simulink model "sampleModel1404"  (R2023a)
settings: Solver=VariableStepAuto  StartTime=0.0  StopTime=10.0  RelTol=1e-3
libraries: simulink x5, hdlsllib x1
settings Model: Creator=user1  LastModifiedBy=user1

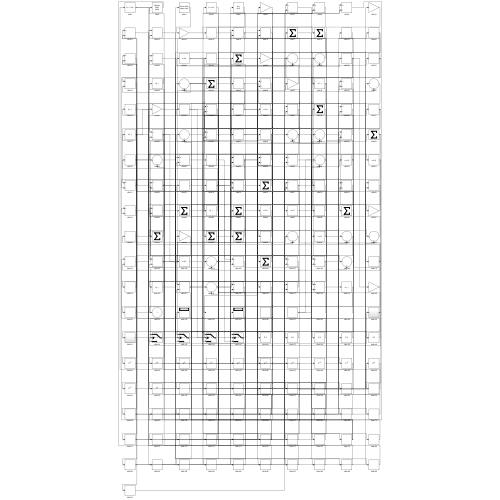
[thumbnail: Simulink's stored preview of the top-level diagram]
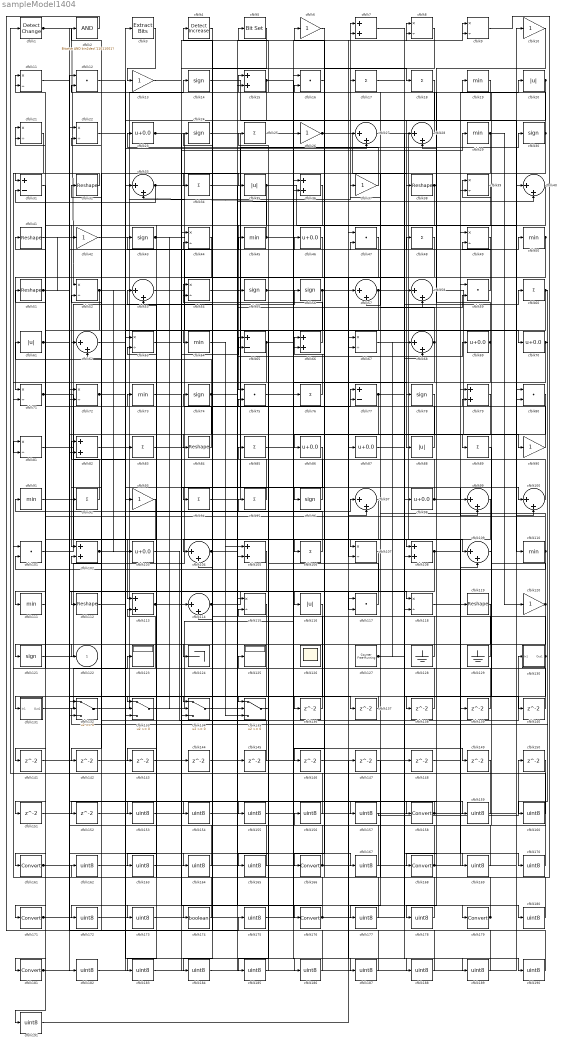
== system sampleModel1404 ==
  cfblk1 : simulink/Logic and Bit Operations/Detect Change  vinit=0  OutDataTypeStr=boolean
      settings: LibrarySourceBlock=|
      | hdlsllib/Logic and Bit
      | Operations/Detect
      | Change
  cfblk{6,10,13,26,37,42,90,93,120} (9 alike) : Gain
  cfblk{27..28,33,40,53,57..58,62,68,97,99..100,104,109,114} (15 alike) : Sum  Inputs=|++
  cfblk{12,16,47,59,75,80,101,117} (8 alike) : DotProduct  OutDataTypeStr=Inherit: Inherit via internal rule
  cfblk{7,15,36,66,79,82,102,105,108,113} (10 alike) : Sum
  cfblk{23,46,69..70,86..87,98,103} (8 alike) : Bias  Bias=0.0  SaturateOnIntegerOverflow=off
  cfblk{17..18,25,34,48,60,76,83,85,89,92,94..95,106} (14 alike) : Sum  Inputs=+
  cfblk{8..9,11,21..22,39,44,49,52,54,63,67,71..72,81,107,115,118} (18 alike) : Product  Inputs=*/  RndMeth=Zero  SaturateOnIntegerOverflow=on
  cfblk{19,29,45,50,64,73,91,110..111} (9 alike) : MinMax
  cfblk{32,38,41,51,84,112,119} (7 alike) : Reshape
  cfblk{20,35,61,88,116} (5 alike) : Abs  SaturateOnIntegerOverflow=off
  cfblk{14,24,30,43,55..56,74,78,96,121} (10 alike) : Signum
  cfblk123 : Display
  cfblk124 : Terminator
  cfblk125 : Display
  cfblk126 : Scope
      settings: Floating=on
  cfblk127 : hdlsllib/Sources/Counter Free-Running  NumBits=16  tsamp=-1
  cfblk128 : Ground
  cfblk129 : Ground
  cfblk130 : Subsystem
      settings: LibrarySourceBlock=|
      | hdlsllib/Ports &
      | Subsystems/Subsystem
  cfblk131 : Subsystem
      settings: LibrarySourceBlock=|
      | hdlsllib/Ports &
      | Subsystems/Subsystem
  cfblk{132..135} (4 alike) : Switch  SaturateOnIntegerOverflow=off  InputSameDT=off
  cfblk{136..152} (17 alike) : Delay  SampleTime=1
  cfblk{153..157,159..160,162..165,167,169..170,172..173,175,177..178,180,182..191} (30 alike) : DataTypeConversion  OutDataTypeStr=uint8  SaturateOnIntegerOverflow=off  RndMeth=Floor
  cfblk{158,161,166,168,171,176,179,181} (8 alike) : DataTypeConversion  SaturateOnIntegerOverflow=off  RndMeth=Floor
  cfblk174 : DataTypeConversion  OutDataTypeStr=boolean  SaturateOnIntegerOverflow=off  RndMeth=Floor
  cfblk2 : simulink/Logic and Bit Operations/Bitwise Operator  logicop=AND  UseBitMask=on  BitMask=bin2dec('11011001')  BitMaskRealWorld=Stored Integer
      settings: LibrarySourceBlock=|
      | hdlsllib/Logic and Bit
      | Operations/Bitwise
      | Operator
  cfblk3 : simulink/Logic and Bit Operations/Extract Bits  bitsToExtract=Upper half  numBits=8  bitIdxRange=[0 7]  outScalingMode=Preserve fixed-point scaling
      settings: LibrarySourceBlock=|
      | hdlsllib/Logic and Bit
      | Operations/Extract Bits
  cfblk31 : Sum  Inputs=+-
  cfblk4 : simulink/Logic and Bit Operations/Detect Increase  vinit=0.0  OutDataTypeStr=boolean
      settings: LibrarySourceBlock=|
      | hdlsllib/Logic and Bit
      | Operations/Detect
      | Increase
  cfblk5 : simulink/Logic and Bit Operations/Bit Set  iBit=0
      settings: LibrarySourceBlock=|
      | hdlsllib/Logic and Bit
      | Operations/Bit Set
  cfblk65 : Sum  Inputs=+-
  cfblk77 : Sum  Inputs=+-
  cfblk122 : Outport  VectorParamsAs1DForOutWhenUnconnected=off
  wires:
  cfblk64/1 -> cfblk105/1
  cfblk93/1 -> cfblk181/1
  cfblk27/1 -> cfblk109/1
  cfblk89/1 -> cfblk135/1
  cfblk79/1 -> cfblk158/1
  cfblk102/1 -> cfblk97/1, cfblk15/2
  cfblk50/1 -> cfblk71/1, cfblk107/2
  cfblk33/1 -> cfblk70/1, cfblk35/1, cfblk31/2, cfblk167/1
  cfblk3/1 -> cfblk13/1
  cfblk18/1 -> cfblk88/1
  cfblk63/1 -> cfblk176/1
  cfblk24/1 -> cfblk100/1
  cfblk84/1 -> cfblk11/1
  cfblk132/1 -> cfblk14/1
  cfblk12/1 -> cfblk83/1
  cfblk54/1 -> cfblk48/1
  cfblk90/1 -> cfblk41/1
  cfblk101/1 -> cfblk56/1
  cfblk103/1 -> cfblk130/1(In1)
  cfblk37/1 -> cfblk23/1
  cfblk118/1 -> cfblk99/1
  cfblk119/1 -> cfblk161/1
  cfblk131/1(Out1) -> cfblk123/1
  cfblk134/1 -> cfblk77/1
  cfblk83/1 -> cfblk50/1
  cfblk58/1 -> cfblk90/1
  cfblk53/1 -> cfblk46/1
  cfblk51/1 -> cfblk42/1, cfblk151/1, cfblk164/1
  cfblk94/1 -> cfblk30/1
  cfblk32/1 -> cfblk31/1
  cfblk38/1 -> cfblk75/1, cfblk108/1
  cfblk65/1 -> cfblk81/2, cfblk104/1, cfblk59/2, cfblk149/1
  cfblk114/1 -> cfblk118/1, cfblk180/1
  cfblk39/1 -> cfblk102/1
  cfblk71/1 -> cfblk113/1, cfblk11/2
  cfblk30/1 -> cfblk118/2, cfblk134/1, cfblk5/1
  cfblk35/1 -> cfblk110/1, cfblk173/1
  cfblk117/1 -> cfblk25/1
  cfblk16/1 -> cfblk106/1
  cfblk81/1 -> cfblk109/2
  cfblk76/1 -> cfblk66/1
  cfblk86/1 -> cfblk133/2
  cfblk26/1 -> cfblk38/1, cfblk146/1
  cfblk97/1 -> cfblk114/2
  cfblk133/1 -> cfblk76/1
  cfblk19/1 -> cfblk96/1
  cfblk109/1 -> cfblk39/1
  cfblk87/1 -> cfblk60/1
  cfblk66/1 -> cfblk54/1
  cfblk42/1 -> cfblk7/1
  cfblk55/1 -> cfblk78/1, cfblk9/2
  cfblk15/1 -> cfblk133/3, cfblk190/1
  cfblk45/1 -> cfblk7/2, cfblk33/2, cfblk108/2
  cfblk21/1 -> cfblk71/2
  cfblk69/1 -> cfblk111/1, cfblk12/2
  cfblk23/1 -> cfblk98/1, cfblk99/2
  cfblk73/1 -> cfblk8/1
  cfblk46/1 -> cfblk121/1
  cfblk121/1 -> cfblk47/1
  cfblk135/1 -> cfblk95/1
  cfblk74/1 -> cfblk69/1, cfblk8/2, cfblk92/1, cfblk135/3, cfblk61/1
  cfblk70/1 -> cfblk132/2, cfblk185/1
  cfblk96/1 -> cfblk24/1
  cfblk92/1 -> cfblk82/1
  cfblk6/1 -> cfblk166/1
  cfblk98/1 -> cfblk20/1, cfblk32/1
  cfblk110/1 -> cfblk75/2, cfblk51/1, cfblk101/2
  cfblk100/1 -> cfblk66/2
  cfblk1/1 -> cfblk52/1, cfblk117/2
  cfblk111/1 -> cfblk21/1
  cfblk107/1 -> cfblk132/3
  cfblk82/1 -> cfblk105/2
  cfblk78/1 -> cfblk86/1
  cfblk85/1 -> cfblk47/2
  cfblk106/1 -> cfblk91/1
  cfblk8/1 -> cfblk116/1
  cfblk29/1 -> cfblk57/2, cfblk112/1, cfblk120/1
  cfblk47/1 -> cfblk122/1
  cfblk68/1 -> cfblk37/1, cfblk143/1
  cfblk127/1 -> cfblk28/1, cfblk68/1
  cfblk17/1 -> cfblk179/1
  cfblk31/1 -> cfblk131/1(In1)
  cfblk13/1 -> cfblk18/1
  cfblk130/1(Out1) -> cfblk19/1, cfblk191/1
  cfblk57/1 -> cfblk140/1, cfblk141/1
  cfblk20/1 -> cfblk28/2, cfblk184/1
  cfblk28/1 -> cfblk15/1
  cfblk129/1 -> cfblk53/1
  cfblk36/1 -> cfblk171/1
  cfblk112/1 -> cfblk27/2
  cfblk95/1 -> cfblk53/2
  cfblk49/1 -> cfblk168/1
  cfblk59/1 -> cfblk55/1
  cfblk43/1 -> cfblk87/1, cfblk134/2
  cfblk56/1 -> cfblk62/1, cfblk9/1, cfblk165/1
  cfblk75/1 -> cfblk89/1
  cfblk77/1 -> cfblk82/2, cfblk68/2
  cfblk5/1 -> cfblk34/1
  cfblk128/1 -> cfblk43/1
  cfblk72/1 -> cfblk135/2, cfblk187/1
  cfblk113/1 -> cfblk65/1, cfblk29/1
  cfblk14/1 -> cfblk100/2
  cfblk48/1 -> cfblk84/1
  cfblk91/1 -> cfblk3/1
  cfblk62/1 -> cfblk64/1
  cfblk120/1 -> cfblk124/1, cfblk77/2
  cfblk60/1 -> cfblk160/1, cfblk174/1
  cfblk4/1 -> cfblk94/1
  cfblk61/1 -> cfblk45/1, cfblk157/1
  cfblk104/1 -> cfblk58/2, cfblk40/2
  cfblk108/1 -> cfblk134/3, cfblk170/1
  cfblk52/1 -> cfblk72/2, cfblk107/1, cfblk103/1
  cfblk88/1 -> cfblk54/2
  cfblk99/1 -> cfblk136/1
  cfblk136/1 -> cfblk72/1
  cfblk11/1 -> cfblk137/1
  cfblk137/1 -> cfblk133/1
  cfblk10/1 -> cfblk138/1
  cfblk138/1 -> cfblk81/1
  cfblk139/1 -> cfblk21/2
  cfblk140/1 -> cfblk113/2
  cfblk141/1 -> cfblk65/2
  cfblk105/1 -> cfblk142/1
  cfblk142/1 -> cfblk114/1
  cfblk143/1 -> cfblk58/1
  cfblk144/1 -> cfblk97/2
  cfblk34/1 -> cfblk145/1
  cfblk145/1 -> cfblk102/2
  cfblk148/1 -> cfblk39/2
  cfblk149/1 -> cfblk1/1
  cfblk151/1 -> cfblk33/1
  cfblk152/1 -> cfblk117/1
  cfblk80/1 -> cfblk153/1
  cfblk153/1 -> cfblk59/1
  cfblk116/1 -> cfblk154/1
  cfblk154/1 -> cfblk80/1
  cfblk155/1 -> cfblk80/2
  cfblk150/1 -> cfblk156/1
  cfblk156/1 -> cfblk52/2
  cfblk157/1 -> cfblk150/1
  cfblk158/1 -> cfblk155/1, cfblk152/1
  cfblk25/1 -> cfblk159/1
  cfblk159/1 -> cfblk79/1
  cfblk160/1 -> cfblk79/2
  cfblk161/1 -> cfblk139/1, cfblk10/1
  cfblk9/1 -> cfblk162/1
  cfblk162/1 -> cfblk119/1
  cfblk44/1 -> cfblk163/1
  cfblk163/1 -> cfblk26/1
  cfblk164/1 -> cfblk44/1
  cfblk165/1 -> cfblk44/2
  cfblk166/1 -> cfblk62/2, cfblk12/1, cfblk85/1
  cfblk167/1 -> cfblk6/1
  cfblk168/1 -> cfblk16/1, cfblk125/1
  cfblk7/1 -> cfblk169/1
  cfblk169/1 -> cfblk49/1
  cfblk170/1 -> cfblk49/2
  cfblk171/1 -> cfblk148/1, cfblk147/1
  cfblk172/1 -> cfblk36/1
  cfblk173/1 -> cfblk36/2
  cfblk174/1 -> cfblk2/1
  cfblk2/1 -> cfblk175/1
  cfblk175/1 -> cfblk27/1
  cfblk176/1 -> cfblk172/1, cfblk101/1, cfblk4/1
  cfblk147/1 -> cfblk177/1
  cfblk177/1 -> cfblk63/1
  cfblk40/1 -> cfblk178/1
  cfblk178/1 -> cfblk63/2
  cfblk179/1 -> cfblk16/2, cfblk104/2, cfblk73/1
  cfblk180/1 -> cfblk17/1
  cfblk181/1 -> cfblk40/1, cfblk57/1
  cfblk41/1 -> cfblk182/1
  cfblk182/1 -> cfblk93/1
  cfblk115/1 -> cfblk183/1
  cfblk183/1 -> cfblk144/1
  cfblk184/1 -> cfblk115/1
  cfblk185/1 -> cfblk115/2
  cfblk22/1 -> cfblk186/1
  cfblk186/1 -> cfblk74/1
  cfblk187/1 -> cfblk22/1
  cfblk146/1 -> cfblk188/1
  cfblk188/1 -> cfblk22/2
  cfblk67/1 -> cfblk189/1
  cfblk189/1 -> cfblk132/1
  cfblk190/1 -> cfblk67/1
  cfblk191/1 -> cfblk67/2

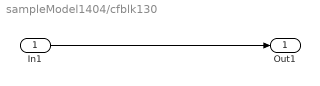
== system sampleModel1404/cfblk130 ==
  In1 : Inport
  Out1 : Outport
  wires:
  In1/1 -> Out1/1

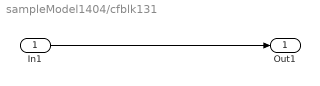
== system sampleModel1404/cfblk131 ==
  In1 : Inport
  Out1 : Outport
  wires:
  In1/1 -> Out1/1
